simulink model "model_with_control"  (R2018a)
settings: Solver=VariableStepAuto  StartTime=0.0  StopTime=35  RelTol=1e-3
values from neighbouring files (symbols this model uses):
  A = [ 0 0 1     0 ... (first row only)    [parameters.m]
  a = len/5    (= 0.1)    [parameters.m]
  B_d = [ 0    0 ... (first row only)    [parameters.m]
  B_u = [ 0   0 ... (first row only)    [parameters.m]
  C_p = [ 1 0 0 0 ... (first row only)    [parameters.m]
  C_s = [ 1 0 0 0 ... (first row only)    [parameters.m]
  f_max = inf    [parameters.m]
  f_min = 0    [parameters.m]
  g = 9.8    [parameters.m]
  K = place(A, B_u, p)    [parameters.m]
  K_i = K_aug(:, 5:6)    [parameters.m]
  K_i_lqr = K_aug_lqr(:, 5:6)    [parameters.m]
  k_r = -inv(C_p*inv(A -B_u*K)*B_u)    [parameters.m]
  k_r_when_K_i = -inv(C_p*inv(A -B_u*K_when_K_i)*B_u)    [parameters.m]
  k_r_when_K_i_lqr = -inv(C_p*inv(A -B_u*K_when_K_i_lqr)*B_u)    [parameters.m]
  K_when_K_i = K_aug(:, 1:4)    [parameters.m]
  K_when_K_i_lqr = K_aug_lqr(:, 1:4)    [parameters.m]
  L = 1    [parameters.m]
  len = .5    (= 0.5)    [parameters.m]
  m = 100    [parameters.m]
libraries: simulink x13
settings Model: Creator=joses  LastModifiedBy=joses
settings SolverCC: ZeroCrossAlgorithm=Adaptive
settings DebuggingCC: MaxConsecutiveZCsMsg=none

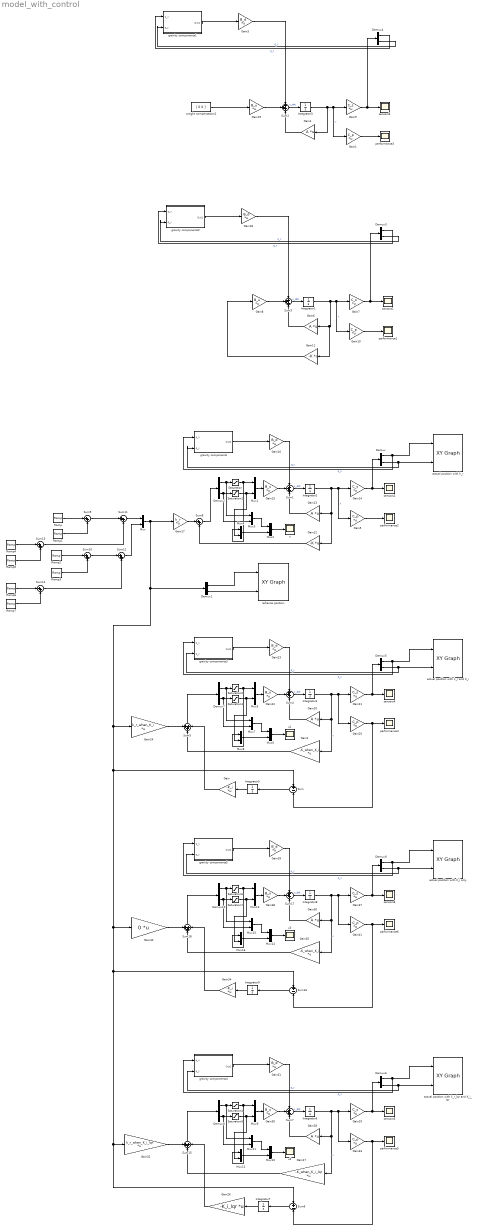
== system model_with_control ==
  Demux{,1..10} (11 alike) : Demux  Outputs=2
  Gain : Gain  Gain=-K_i  Multiplication=Matrix(K*u)
  Gain{1,5,10,25,33,41} (6 alike) : Gain  Gain=C_p  Multiplication=Matrix(K*u)
  Gain11 : Gain  Gain=-K  Multiplication=Matrix(K*u)
  Gain12 : Gain  Gain=-K  Multiplication=Matrix(K*u)
  Gain{4,6,13,20,28,36} (6 alike) : Gain  Gain=A  Multiplication=Matrix(K*u)
  Gain{7,9,14,21,29,37} (6 alike) : Gain  Gain=C_s  Multiplication=Matrix(K*u)
  Gain{8,15,19,22,30,38} (6 alike) : Gain  Gain=B_u  Multiplication=Matrix(K*u)
  Gain{3,16,18,23,31,39} (6 alike) : Gain  Gain=B_d  Multiplication=Matrix(K*u)
  Gain17 : Gain  Gain=k_r  Multiplication=Matrix(K*u)
  Gain2 : Gain  Gain=-K_when_K_i  Multiplication=Matrix(K*u)
  Gain24 : Gain  Gain=k_r_when_K_i  Multiplication=Matrix(K*u)
  Gain26 : Gain  Gain=-K_i_lqr  Multiplication=Matrix(K*u)
  Gain27 : Gain  Gain=-K_when_K_i_lqr  Multiplication=Matrix(K*u)
  Gain32 : Gain  Gain=k_r_when_K_i_lqr  Multiplication=Matrix(K*u)
  Gain34 : Gain  Gain=-K_i  Multiplication=Matrix(K*u)
  Gain35 : Gain  Gain=-K_when_K_i  Multiplication=Matrix(K*u)
  Gain40 : Gain  Gain=0  Multiplication=Matrix(K*u)
  Integrator{1..4,6,8} (6 alike) : Integrator  InitialCondition=[0,0,0,0]'
  Integrator5 : Integrator  InitialCondition=[0,0]'
  Integrator7 : Integrator  InitialCondition=[0,0]'
  Integrator9 : Integrator  InitialCondition=[0,0]'
  Mux{,1..16} (17 alike) : Mux  Inputs=2
  Ramp : simulink/Sources/Ramp  slope=a  start=10  InitialOutput=0
  Ramp1 : simulink/Sources/Ramp  slope=-a  start=15  InitialOutput=0
  Ramp2 : simulink/Sources/Ramp  slope=a  start=15  InitialOutput=0
  Ramp3 : simulink/Sources/Ramp  slope=-a  start=20  InitialOutput=0
  Ramp4 : simulink/Sources/Ramp  slope=-a  start=20  InitialOutput=0
  Ramp5 : simulink/Sources/Ramp  slope=a  start=25  InitialOutput=0
  Ramp6 : simulink/Sources/Ramp  slope=-a  start=25  InitialOutput=0
  Ramp7 : simulink/Sources/Ramp  slope=a  start=30  InitialOutput=0
  Saturation{,1..7} (8 alike) : Saturate  UpperLimit=f_max  LowerLimit=f_min
  Sum : Sum  Inputs=+-
  Sum{1..5,7,15,17..18} (9 alike) : Sum  Inputs=+++
  Sum{8..14} (7 alike) : Sum  Inputs=|++
  Sum16 : Sum  Inputs=+-
  Sum6 : Sum  Inputs=+-
  actual position with K_i only : simulink/Sinks/XY Graph  xmin=-1  xmax=2*len  ymin=-1  ymax=2*len  st=-1
  actual position with k_r : simulink/Sinks/XY Graph  xmin=-1  xmax=2*len  ymin=-1  ymax=2*len  st=-1
  actual position with k_r and K_i : simulink/Sinks/XY Graph  xmin=-1  xmax=2*len  ymin=-1  ymax=2*len  st=-1
  actual position with k_r_lqr and K_i_lqr : simulink/Sinks/XY Graph  xmin=-1  xmax=2*len  ymin=-1  ymax=2*len  st=-1
  gravity components : Subsystem
  gravity components1 : Subsystem
  gravity components2 : Subsystem
  gravity components3 : Subsystem
  gravity components4 : Subsystem
  gravity components5 : Subsystem
  performance{1..6} (6 alike) : Scope
  refrence position : simulink/Sinks/XY Graph  xmin=-1  xmax=2*len  ymin=-1  ymax=2*len  st=-1
  sensors{1..6} (6 alike) : Scope
  u{,1..3} (4 alike) : Scope
  weight compensation2 : Constant  Value=[ 0 0 ]'
  wires:
  Gain10/1 -> performance1/1
  Gain6/1 -> Sum3/3
  Sum3/1 -> Integrator1/1  "x_dot"
  Integrator1/1 -> Gain11/1, Gain6/1, Gain10/1, Gain7/1  "x"
  Gain18/1 -> Sum3/1
  Gain11/1 -> Gain8/1
  Gain8/1 -> Sum3/2
  Gain12/1 -> Sum8/2
  Sum1/1 -> Integrator2/1  "x_dot"
  Gain13/1 -> Sum1/3
  Gain14/1 -> Demux/1, sensors2/1
  Gain5/1 -> performance2/1
  Integrator2/1 -> Gain12/1, Gain13/1, Gain5/1, Gain14/1  "x"
  Gain17/1 -> Sum8/1
  Ramp/1 -> Sum9/1
  Sum9/1 -> Sum11/1
  Ramp1/1 -> Sum9/2
  Ramp2/1 -> Sum10/1
  Ramp3/1 -> Sum10/2
  Sum11/1 -> Mux/1
  Sum10/1 -> Sum12/1
  Sum12/1 -> Mux/2
  Ramp4/1 -> Sum13/1
  Ramp5/1 -> Sum13/2
  Sum13/1 -> Sum11/2
  Ramp7/1 -> Sum14/2
  Sum14/1 -> Sum12/2
  Ramp6/1 -> Sum14/1
  Demux/1 -> gravity components/1(q_x), actual position with k_r/1  "q_x"
  Demux/2 -> gravity components/2(q_y), actual position with k_r/2  "q_y"
  Demux1/2 -> refrence position/2
  Demux1/1 -> refrence position/1
  Mux1/1 -> Gain15/1
  Sum8/1 -> Demux2/1
  Saturation/1 -> Mux4/1, Mux1/1
  Saturation1/1 -> Mux4/2, Mux1/2
  Demux2/2 -> Mux3/2, Saturation1/1
  Mux2/1 -> u/1
  Demux2/1 -> Mux3/1, Saturation/1
  Gain15/1 -> Sum1/2
  gravity components/1(Out1) -> Gain16/1
  Mux3/1 -> Mux2/1
  Mux4/1 -> Mux2/2
  Gain16/1 -> Sum1/1
  gravity components2/1(Out1) -> Gain18/1
  Gain7/1 -> Demux3/1, sensors1/1
  Demux3/2 -> gravity components2/2(q_y)  "q_y"
  Demux3/1 -> gravity components2/1(q_x)  "q_x"
  Demux4/1 -> gravity components1/1(q_x)  "q_x"
  Demux4/2 -> gravity components1/2(q_y)  "q_y"
  gravity components1/1(Out1) -> Gain3/1
  Sum2/1 -> Integrator3/1  "x_dot"
  Gain4/1 -> Sum2/3
  weight compensation2/1 -> Gain19/1
  Gain1/1 -> performance3/1
  Integrator3/1 -> Gain4/1, Gain1/1, Gain9/1  "x"
  Gain9/1 -> Demux4/1, sensors3/1
  Gain3/1 -> Sum2/1
  Gain19/1 -> Sum2/2
  gravity components3/1(Out1) -> Gain23/1
  Gain21/1 -> Demux5/1, sensors4/1
  Sum4/1 -> Integrator4/1  "x_dot"
  Sum5/1 -> Demux7/1
  Mux6/1 -> u1/1
  Mux7/1 -> Mux6/1
  Gain23/1 -> Sum4/1
  Saturation2/1 -> Mux8/1, Mux5/1
  Integrator4/1 -> Gain2/1, Gain20/1, Gain25/1, Gain21/1  "x"
  Gain24/1 -> Sum5/1
  Gain2/1 -> Sum5/2
  Mux5/1 -> Gain22/1
  Demux5/2 -> gravity components3/2(q_y), actual position with k_r and K_i/2  "q_y"
  Gain22/1 -> Sum4/2
  Demux7/2 -> Mux7/2, Saturation3/1
  Gain25/1 -> Sum/2, performance4/1
  Mux8/1 -> Mux6/2
  Demux5/1 -> gravity components3/1(q_x), actual position with k_r and K_i/1  "q_x"
  Gain20/1 -> Sum4/3
  Saturation3/1 -> Mux8/2, Mux5/2
  Demux7/1 -> Mux7/1, Saturation2/1
  Sum/1 -> Integrator5/1
  Integrator5/1 -> Gain/1
  Gain/1 -> Sum5/3
  Sum6/1 -> Integrator7/1
  Demux8/1 -> Mux11/1, Saturation4/1
  Saturation5/1 -> Mux12/2, Mux9/2
  Mux/1 -> Demux1/1, Sum6/1, Gain32/1, Sum16/1, Gain40/1, Sum/1, Gain24/1, Gain17/1
  Gain30/1 -> Sum7/2
  Demux8/2 -> Mux11/2, Saturation5/1
  Gain32/1 -> Sum15/1
  Gain26/1 -> Sum15/3
  Gain27/1 -> Sum15/2
  Integrator6/1 -> Gain27/1, Gain28/1, Gain33/1, Gain29/1  "x"
  Demux6/2 -> gravity components4/2(q_y), actual position with k_r_lqr and K_i_lqr/2  "q_y"
  Gain33/1 -> Sum6/2, performance5/1
  Mux12/1 -> Mux10/2
  Saturation4/1 -> Mux12/1, Mux9/1
  Demux6/1 -> gravity components4/1(q_x), actual position with k_r_lqr and K_i_lqr/1  "q_x"
  Mux11/1 -> Mux10/1
  Mux10/1 -> u2/1
  Mux9/1 -> Gain30/1
  Gain28/1 -> Sum7/3
  Sum15/1 -> Demux8/1
  Gain29/1 -> Demux6/1, sensors5/1
  Gain31/1 -> Sum7/1
  Sum7/1 -> Integrator6/1  "x_dot"
  Integrator7/1 -> Gain26/1
  gravity components4/1(Out1) -> Gain31/1
  Sum16/1 -> Integrator9/1
  Demux10/1 -> Mux15/1, Saturation6/1
  Saturation7/1 -> Mux16/2, Mux13/2
  Gain38/1 -> Sum17/2
  Demux10/2 -> Mux15/2, Saturation7/1
  Gain40/1 -> Sum18/1
  Gain34/1 -> Sum18/3
  Gain35/1 -> Sum18/2
  Integrator8/1 -> Gain35/1, Gain36/1, Gain41/1, Gain37/1  "x"
  Demux9/2 -> gravity components5/2(q_y), actual position with K_i only/2  "q_y"
  Gain41/1 -> Sum16/2, performance6/1
  Mux16/1 -> Mux14/2
  Saturation6/1 -> Mux16/1, Mux13/1
  Demux9/1 -> gravity components5/1(q_x), actual position with K_i only/1  "q_x"
  Mux15/1 -> Mux14/1
  Mux14/1 -> u3/1
  Mux13/1 -> Gain38/1
  Gain36/1 -> Sum17/3
  Sum18/1 -> Demux10/1
  Gain37/1 -> Demux9/1, sensors6/1
  Gain39/1 -> Sum17/1
  Sum17/1 -> Integrator8/1  "x_dot"
  Integrator9/1 -> Gain34/1
  gravity components5/1(Out1) -> Gain39/1

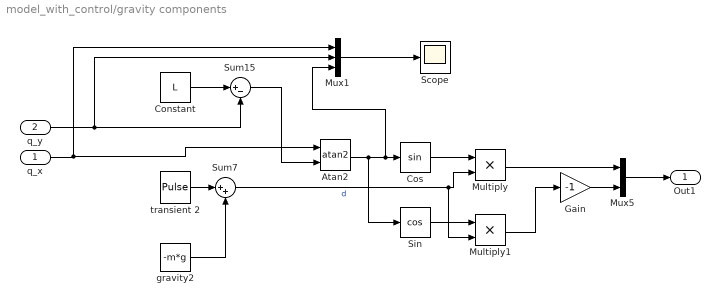
== system model_with_control/gravity components ==
  q_x : Inport
  q_y : Inport  Port=2
  Atan2 : Trigonometry  Operator=atan2
  Constant : Constant  Value=L
  Cos : Trigonometry
  Gain : Gain  Gain=-1
  Multiply : Product
  Multiply1 : Product
  Mux1 : Mux  Inputs=3
  Mux5 : Mux  Inputs=2
  Scope : Scope
  Sin : Trigonometry  Operator=cos
  Sum15 : Sum  Inputs=|+-
  Sum7 : Sum  Inputs=|++
  gravity2 : Constant  Value=-m*g
  transient 2 : DiscretePulseGenerator  PulseType=Time based  Amplitude=-m*g  Period=500  PulseWidth=1/5  PhaseDelay=5
  Out1 : Outport
  wires:
  Sum7/1 -> Multiply1/2, Multiply/2  "d"
  Multiply1/1 -> Gain/1
  Sin/1 -> Multiply1/1
  Cos/1 -> Multiply/1
  Constant/1 -> Sum15/1
  Atan2/1 -> Sin/1, Mux1/3, Cos/1
  gravity2/1 -> Sum7/2
  transient 2/1 -> Sum7/1
  Multiply/1 -> Mux5/1
  Mux5/1 -> Out1/1
  q_y/1 -> Mux1/2, Sum15/2
  q_x/1 -> Atan2/1, Mux1/1
  Mux1/1 -> Scope/1
  Sum15/1 -> Atan2/2
  Gain/1 -> Mux5/2

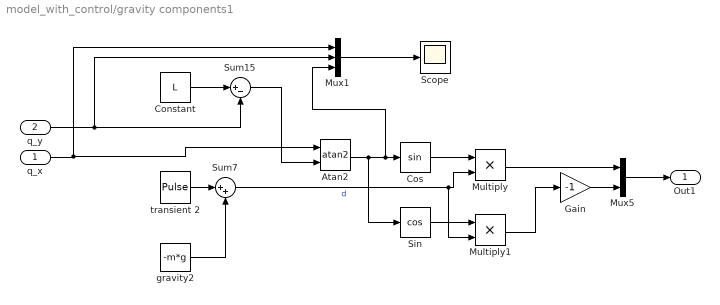
== system model_with_control/gravity components1 ==
  q_x : Inport
  q_y : Inport  Port=2
  Atan2 : Trigonometry  Operator=atan2
  Constant : Constant  Value=L
  Cos : Trigonometry
  Gain : Gain  Gain=-1
  Multiply : Product
  Multiply1 : Product
  Mux1 : Mux  Inputs=3
  Mux5 : Mux  Inputs=2
  Scope : Scope
  Sin : Trigonometry  Operator=cos
  Sum15 : Sum  Inputs=|+-
  Sum7 : Sum  Inputs=|++
  gravity2 : Constant  Value=-m*g
  transient 2 : DiscretePulseGenerator  PulseType=Time based  Amplitude=-m*g  Period=500  PulseWidth=1/5  PhaseDelay=5
  Out1 : Outport
  wires:
  Sum7/1 -> Multiply1/2, Multiply/2  "d"
  Multiply1/1 -> Gain/1
  Sin/1 -> Multiply1/1
  Cos/1 -> Multiply/1
  Constant/1 -> Sum15/1
  Atan2/1 -> Sin/1, Mux1/3, Cos/1
  gravity2/1 -> Sum7/2
  transient 2/1 -> Sum7/1
  Multiply/1 -> Mux5/1
  Mux5/1 -> Out1/1
  q_y/1 -> Mux1/2, Sum15/2
  q_x/1 -> Atan2/1, Mux1/1
  Mux1/1 -> Scope/1
  Sum15/1 -> Atan2/2
  Gain/1 -> Mux5/2

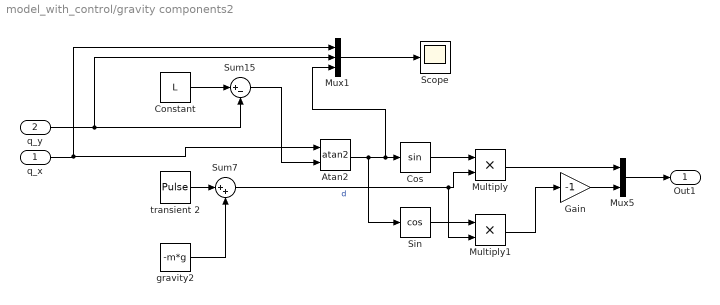
== system model_with_control/gravity components2 ==
  q_x : Inport
  q_y : Inport  Port=2
  Atan2 : Trigonometry  Operator=atan2
  Constant : Constant  Value=L
  Cos : Trigonometry
  Gain : Gain  Gain=-1
  Multiply : Product
  Multiply1 : Product
  Mux1 : Mux  Inputs=3
  Mux5 : Mux  Inputs=2
  Scope : Scope
  Sin : Trigonometry  Operator=cos
  Sum15 : Sum  Inputs=|+-
  Sum7 : Sum  Inputs=|++
  gravity2 : Constant  Value=-m*g
  transient 2 : DiscretePulseGenerator  PulseType=Time based  Amplitude=-m*g  Period=500  PulseWidth=1/5  PhaseDelay=5
  Out1 : Outport
  wires:
  Sum7/1 -> Multiply1/2, Multiply/2  "d"
  Multiply1/1 -> Gain/1
  Sin/1 -> Multiply1/1
  Cos/1 -> Multiply/1
  Constant/1 -> Sum15/1
  Atan2/1 -> Sin/1, Mux1/3, Cos/1
  gravity2/1 -> Sum7/2
  transient 2/1 -> Sum7/1
  Multiply/1 -> Mux5/1
  Mux5/1 -> Out1/1
  q_y/1 -> Mux1/2, Sum15/2
  q_x/1 -> Atan2/1, Mux1/1
  Mux1/1 -> Scope/1
  Sum15/1 -> Atan2/2
  Gain/1 -> Mux5/2

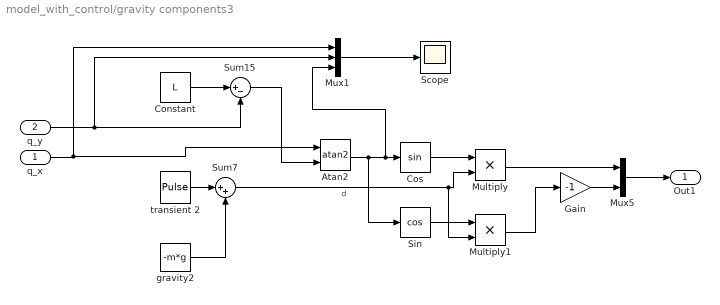
== system model_with_control/gravity components3 ==
  q_x : Inport
  q_y : Inport  Port=2
  Atan2 : Trigonometry  Operator=atan2
  Constant : Constant  Value=L
  Cos : Trigonometry
  Gain : Gain  Gain=-1
  Multiply : Product
  Multiply1 : Product
  Mux1 : Mux  Inputs=3
  Mux5 : Mux  Inputs=2
  Scope : Scope
  Sin : Trigonometry  Operator=cos
  Sum15 : Sum  Inputs=|+-
  Sum7 : Sum  Inputs=|++
  gravity2 : Constant  Value=-m*g
  transient 2 : DiscretePulseGenerator  PulseType=Time based  Amplitude=-m*g  Period=500  PulseWidth=1/5  PhaseDelay=5
  Out1 : Outport
  wires:
  Sum7/1 -> Multiply1/2, Multiply/2  "d"
  Multiply1/1 -> Gain/1
  Sin/1 -> Multiply1/1
  Cos/1 -> Multiply/1
  Constant/1 -> Sum15/1
  Atan2/1 -> Sin/1, Mux1/3, Cos/1
  gravity2/1 -> Sum7/2
  transient 2/1 -> Sum7/1
  Multiply/1 -> Mux5/1
  Mux5/1 -> Out1/1
  q_y/1 -> Mux1/2, Sum15/2
  q_x/1 -> Atan2/1, Mux1/1
  Mux1/1 -> Scope/1
  Sum15/1 -> Atan2/2
  Gain/1 -> Mux5/2

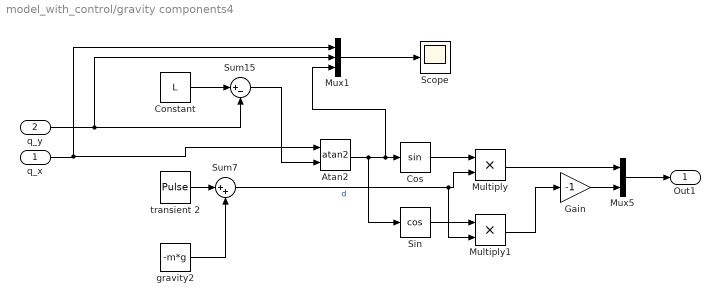
== system model_with_control/gravity components4 ==
  q_x : Inport
  q_y : Inport  Port=2
  Atan2 : Trigonometry  Operator=atan2
  Constant : Constant  Value=L
  Cos : Trigonometry
  Gain : Gain  Gain=-1
  Multiply : Product
  Multiply1 : Product
  Mux1 : Mux  Inputs=3
  Mux5 : Mux  Inputs=2
  Scope : Scope
  Sin : Trigonometry  Operator=cos
  Sum15 : Sum  Inputs=|+-
  Sum7 : Sum  Inputs=|++
  gravity2 : Constant  Value=-m*g
  transient 2 : DiscretePulseGenerator  PulseType=Time based  Amplitude=-m*g  Period=500  PulseWidth=1/5  PhaseDelay=5
  Out1 : Outport
  wires:
  Sum7/1 -> Multiply1/2, Multiply/2  "d"
  Multiply1/1 -> Gain/1
  Sin/1 -> Multiply1/1
  Cos/1 -> Multiply/1
  Constant/1 -> Sum15/1
  Atan2/1 -> Sin/1, Mux1/3, Cos/1
  gravity2/1 -> Sum7/2
  transient 2/1 -> Sum7/1
  Multiply/1 -> Mux5/1
  Mux5/1 -> Out1/1
  q_y/1 -> Mux1/2, Sum15/2
  q_x/1 -> Atan2/1, Mux1/1
  Mux1/1 -> Scope/1
  Sum15/1 -> Atan2/2
  Gain/1 -> Mux5/2

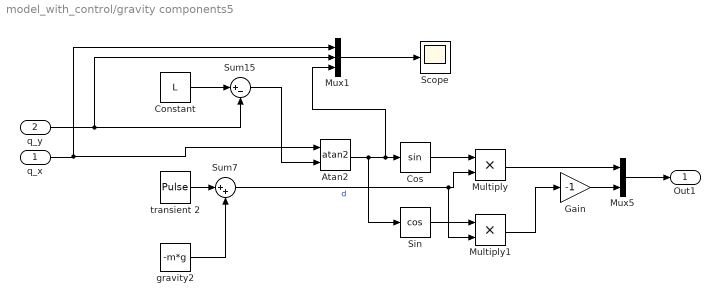
== system model_with_control/gravity components5 ==
  q_x : Inport
  q_y : Inport  Port=2
  Atan2 : Trigonometry  Operator=atan2
  Constant : Constant  Value=L
  Cos : Trigonometry
  Gain : Gain  Gain=-1
  Multiply : Product
  Multiply1 : Product
  Mux1 : Mux  Inputs=3
  Mux5 : Mux  Inputs=2
  Scope : Scope
  Sin : Trigonometry  Operator=cos
  Sum15 : Sum  Inputs=|+-
  Sum7 : Sum  Inputs=|++
  gravity2 : Constant  Value=-m*g
  transient 2 : DiscretePulseGenerator  PulseType=Time based  Amplitude=-m*g  Period=500  PulseWidth=1/5  PhaseDelay=5
  Out1 : Outport
  wires:
  Sum7/1 -> Multiply1/2, Multiply/2  "d"
  Multiply1/1 -> Gain/1
  Sin/1 -> Multiply1/1
  Cos/1 -> Multiply/1
  Constant/1 -> Sum15/1
  Atan2/1 -> Sin/1, Mux1/3, Cos/1
  gravity2/1 -> Sum7/2
  transient 2/1 -> Sum7/1
  Multiply/1 -> Mux5/1
  Mux5/1 -> Out1/1
  q_y/1 -> Mux1/2, Sum15/2
  q_x/1 -> Atan2/1, Mux1/1
  Mux1/1 -> Scope/1
  Sum15/1 -> Atan2/2
  Gain/1 -> Mux5/2
